simulink model "Simple_flight_around_ground_target__Sim"  (R2025b)
settings: Solver=FixedStepAuto  StartTime=0.0  StopTime=10  FixedStep=1/2000  RelTol=1e-3
undefined symbols (not defined in the file or in its folder): nFrames, pitchVec, yawVec
libraries: simulink_extras x7, MISSILE_GUIDANCE_LIB2 x5, simulink x2
settings Model: NumberOfSteps=50  PacingRate=0.011000  Creator=Leonid  LastModifiedBy=Leonid

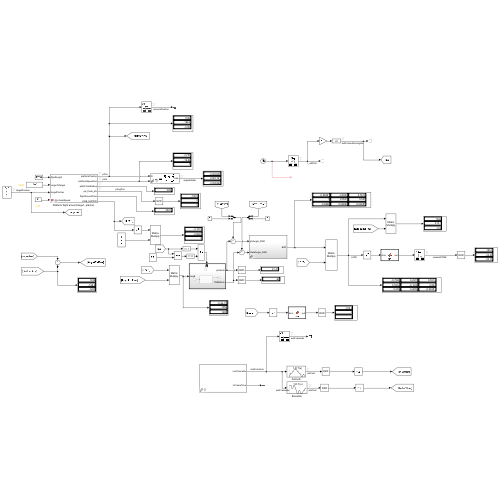
[thumbnail: Simulink's stored preview of the top-level diagram]
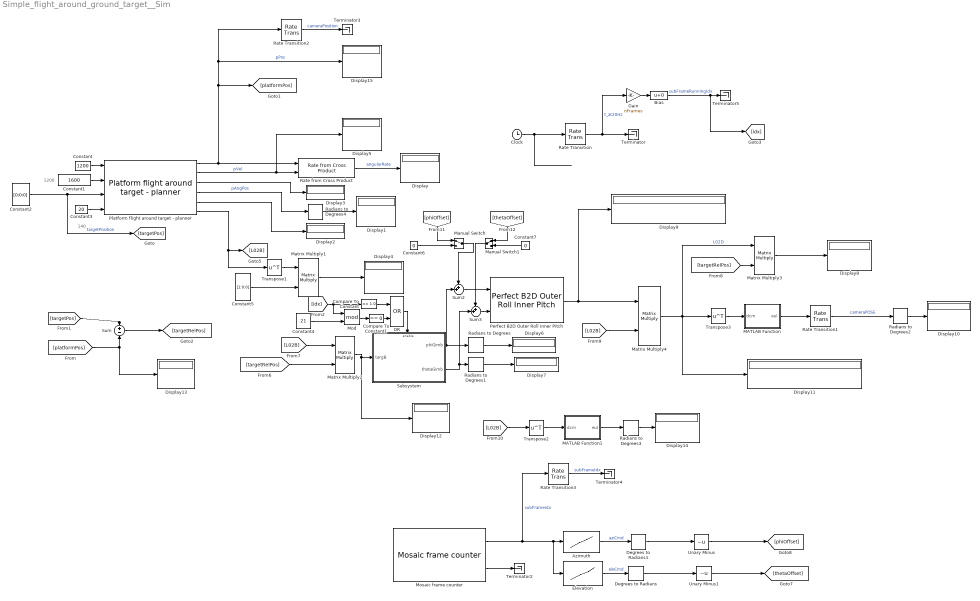
== system Simple_flight_around_ground_target__Sim ==
  note: 140
  note: 1200
  Azimuth : Lookup_n-D  NumberOfTableDimensions=1  BreakpointsForDimension1=1:nFrames  Table=yawVec  InternalRulePriority=Speed  RndMeth=Simplest
  Bias : Bias  SaturateOnIntegerOverflow=off
  Clock : Clock
  Compare To Constant : simulink/Logic and Bit Operations/Compare To Constant  relop===  const=1.0  OutDataTypeStr=boolean
  Compare To Constant1 : simulink/Logic and Bit Operations/Compare To Constant  relop===  const=0  OutDataTypeStr=boolean
  Constant : Constant  Value=1200
  Constant1 : Constant  Value=1600
  Constant2 : Constant  Value=[0;0;0]  VectorParams1D=off
  Constant3 : Constant  Value=20
  Constant4 : Constant  Value=21
  Constant5 : Constant  Value=[1;0;0]  VectorParams1D=off
  Constant6 : Constant  Value=0
  Constant7 : Constant  Value=0
  Degrees to Radians : simulink_extras/Transformations/Degrees to Radians
  Degrees to Radians1 : simulink_extras/Transformations/Degrees to Radians
  Display{,1..15} (16 alike) : Display
  Elevation : Lookup_n-D  NumberOfTableDimensions=1  BreakpointsForDimension1=1:nFrames  Table=pitchVec  InternalRulePriority=Speed  RndMeth=Simplest
  Gain : Gain  Gain=nFrames
  MATLAB Function : MATLAB Function  TreatAsAtomicUnit=on
  MATLAB Function1 : MATLAB Function  TreatAsAtomicUnit=on
  Manual Switch : ManualSwitch
  Manual Switch1 : ManualSwitch
  Matrix Multiply{1..4} (4 alike) : Product  Multiplication=Matrix(*)
  Mod : Math  Operator=mod
  Mosaic frame counter : MISSILE_GUIDANCE_LIB2/Mosaic frame counter  nFrames=20
  OR : Logic  Operator=OR  AllPortsSameDT=off  OutDataTypeStr=boolean
  Perfect B2D Outer Roll Inner Pitch : MISSILE_GUIDANCE_LIB2/Perfect B2D Outer Roll Inner Pitch  SystemSampleTime=-1  VariantActivationTime=update diagram  EmptyChoice=off  PassThrough=off  PassThroughVariantControl=(default)  EmptyChoiceVariantControl=(default)  AllowFlexibleInterface=on  Latency=0  AutoFrameSizeCalculation=off
  "Platform flight around target - planner " : MISSILE_GUIDANCE_LIB2/Platform flight around target - planner   fs=10000  psi0_theta0_phi0=[90:0:0]
      link override quaternion Integration1: ts=1/2000  psi0_theta0_phi0=[-90;0;0]
  Radians to Degrees{,1..4} (5 alike) : simulink_extras/Transformations/Radians to Degrees
  Rate Transition : RateTransition  OutPortSampleTime=1/nFrames
  Rate Transition1 : RateTransition  OutPortSampleTime=1/20
  Rate Transition2 : RateTransition  OutPortSampleTime=1/20
  Rate Transition3 : RateTransition  OutPortSampleTime=1/nFrames
  Rate from Cross Product : MISSILE_GUIDANCE_LIB2/Rate from Cross Product
  Subsystem : Subsystem
  Sum : Sum  Inputs=+|-
  Sum2 : Sum  Inputs=++|
  Sum3 : Sum  Inputs=++|
  Terminator{,2..5} (5 alike) : Terminator
  Transpose1 : Math  Operator=transpose
  Transpose2 : Math  Operator=transpose
  Transpose3 : Math  Operator=transpose
  Unary Minus : UnaryMinus
  Unary Minus1 : UnaryMinus
  wires:
  Constant/1 -> "Platform flight around target - planner "/1
  Constant1/1 -> "Platform flight around target - planner "/2
  Constant2/1 -> [targetPos], "Platform flight around target - planner "/3  "targetPosition"
  Constant3/1 -> "Platform flight around target - planner "/4
  Rate from Cross Product/1 -> Display/1  "angularRate"
  "Platform flight around target - planner "/4 -> Radians to Degrees4/1  "pAngPos"
  "Platform flight around target - planner "/5 -> Display2/1
  "Platform flight around target - planner "/3 -> Display3/1
  "Platform flight around target - planner "/1 -> Display15/1, Rate Transition2/1, [platformPos], Rate from Cross Product/1  "pPos"
  "Platform flight around target - planner "/6 -> [L02B], Transpose1/1
  Constant5/1 -> Matrix Multiply1/2
  Matrix Multiply1/1 -> Display4/1
  Transpose1/1 -> Matrix Multiply1/1
  "Platform flight around target - planner "/2 -> Rate from Cross Product/2, Display5/1  "pVel"
  [targetPos] -> Sum/1
  [platformPos] -> Display13/1, Sum/2
  Sum/1 -> [targetRelPos]
  [targetRelPos] -> Matrix Multiply2/2
  Radians to Degrees/1 -> Display6/1
  Radians to Degrees1/1 -> Display7/1
  [L02B] -> Matrix Multiply2/1
  Matrix Multiply2/1 -> Subsystem/1(targB), Display12/1
  Perfect B2D Outer Roll Inner Pitch/1 -> Display9/1, Matrix Multiply4/1
  [L02B] -> Matrix Multiply4/2
  Matrix Multiply4/1 -> Transpose3/1, Display11/1, Matrix Multiply3/1  "L02D"
  [targetRelPos] -> Matrix Multiply3/2
  Matrix Multiply3/1 -> Display8/1
  Radians to Degrees2/1 -> Display10/1
  [L02B] -> Transpose2/1
  MATLAB Function1/1(eul) -> Radians to Degrees3/1
  Radians to Degrees3/1 -> Display14/1
  Transpose2/1 -> MATLAB Function1/1(dcm)
  Transpose3/1 -> MATLAB Function/1(dcm)
  Clock/1 -> Rate Transition/1
  Rate Transition/1 -> Gain/1, Terminator/1  "t_at20Hz"
  Mosaic frame counter/1 -> Rate Transition3/1, Elevation/1, Azimuth/1  "subFrameIdx"
  Mosaic frame counter/2 -> Terminator2/1
  Azimuth/1 -> Degrees to Radians1/1  "aziCmd"
  Elevation/1 -> Degrees to Radians/1  "eleCmd"
  Sum2/1 -> Perfect B2D Outer Roll Inner Pitch/1
  Sum3/1 -> Perfect B2D Outer Roll Inner Pitch/2
  [phiOffset] -> Manual Switch/1
  [thetaOffset] -> Manual Switch1/1
  Manual Switch/1 -> Sum2/1
  Manual Switch1/1 -> Sum3/1
  Constant6/1 -> Manual Switch/2
  Constant7/1 -> Manual Switch1/2
  Radians to Degrees4/1 -> Display1/1
  MATLAB Function/1(eul) -> Rate Transition1/1
  Rate Transition1/1 -> Radians to Degrees2/1  "cameraPOSE"
  Rate Transition2/1 -> Terminator3/1  "cameraPosition"
  Rate Transition3/1 -> Terminator4/1  "subFrameIdx"
  Degrees to Radians1/1 -> Unary Minus/1
  Degrees to Radians/1 -> Unary Minus1/1
  Gain/1 -> Bias/1
  Unary Minus/1 -> [phiOffset]
  Unary Minus1/1 -> [thetaOffset]
  Bias/1 -> [idx], Terminator5/1  "subFrameRunningIdx"
  [idx] -> Compare To Constant/1, Mod/1
  Compare To Constant/1 -> OR/1
  Constant4/1 -> Mod/2
  Mod/1 -> Compare To Constant1/1
  OR/1 -> Subsystem/Enable
  Subsystem/1(phiGimb) -> Sum2/2, Radians to Degrees/1
  Subsystem/2(thetaGimb) -> Sum3/2, Radians to Degrees1/1
  Compare To Constant1/1 -> OR/2

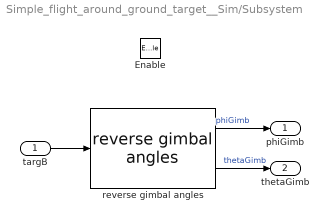
== system Simple_flight_around_ground_target__Sim/Subsystem ==
  targB : Inport
  Enable : EnablePort
  reverse gimbal angles : MISSILE_GUIDANCE_LIB2/reverse gimbal angles  SystemSampleTime=-1  VariantActivationTime=update diagram  EmptyChoice=off  PassThrough=off  PassThroughVariantControl=(default)  EmptyChoiceVariantControl=(default)  AllowFlexibleInterface=on  Latency=0  AutoFrameSizeCalculation=off
  phiGimb : Outport
  thetaGimb : Outport  Port=2
  wires:
  reverse gimbal angles/1 -> phiGimb/1  "phiGimb"
  targB/1 -> reverse gimbal angles/1
  reverse gimbal angles/2 -> thetaGimb/1  "thetaGimb"

== matlab function Simple_flight_around_ground_target__Sim/MATLAB Function ==
  data: dcm input; eul output
function eul = fcn(dcm)

eul = rotm2eul(dcm);

== matlab function Simple_flight_around_ground_target__Sim/MATLAB Function1 ==
  data: dcm input; eul output
function eul = fcn(dcm)

eul = rotm2eul(dcm);
